simulink model "Saturation_subsystem_in_Mask"  (R2022b)
settings: Solver=FixedStepDiscrete  StartTime=0.0  StopTime=10.0  FixedStep=1e-3  RelTol=1e-3
settings Model: Creator=Abanob_Sameh  LastModifiedBy=Abanob_Sameh

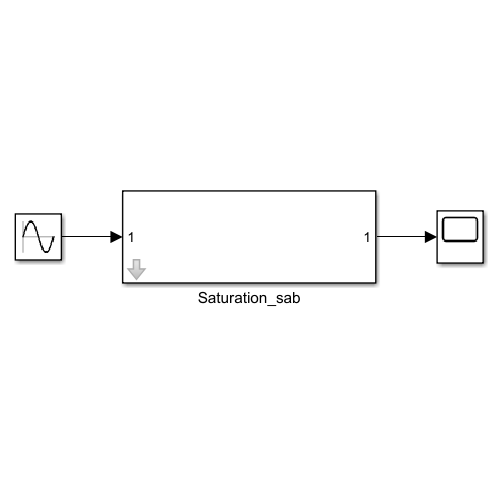
[thumbnail: Simulink's stored preview of the top-level diagram]
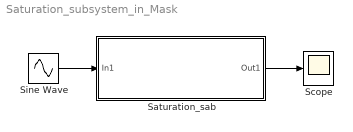
== system Saturation_subsystem_in_Mask ==
  Saturation_sab : Subsystem  mask{u=0.5, L=0.5}
      mask prompts: u "Upper limit:"; L "Lower limit:"
  Scope : Scope
  Sine Wave : Sin  SampleTime=0
  wires:
  Sine Wave/1 -> Saturation_sab/1(In1)
  Saturation_sab/1(Out1) -> Scope/1

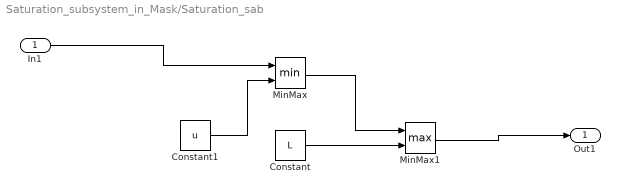
== system Saturation_subsystem_in_Mask/Saturation_sab ==
  In1 : Inport
  Constant : Constant  Value=L
  Constant1 : Constant  Value=u
  MinMax : MinMax  Inputs=2  ZeroCross=off
  MinMax1 : MinMax  Function=max  Inputs=2
  Out1 : Outport
  wires:
  MinMax1/1 -> Out1/1
  MinMax/1 -> MinMax1/1
  Constant/1 -> MinMax1/2
  In1/1 -> MinMax/1
  Constant1/1 -> MinMax/2
